simulink model "kinematics"  (R2019a)
settings: Solver=ode45  StartTime=0.0  StopTime=60  RelTol=2.8421709430404007E-14
undefined symbols (not defined in the file or in its folder): A0_BI, q0_BI, theta0_BI, wbi0_B, X, Y, Z, zyx0
libraries: sm_lib x3, nesl_utility x1
settings Model: Creator=bbingham  LastModifiedBy=tjones
settings DataIOCC: ReturnWorkspaceOutputs=off
settings DebuggingCC: ArithmeticOperatorsInVariantConditions=warning
settings SFSimCC: SimUseLocalCustomCode=off
settings RTWCC: SystemTargetFile=sldrt.tlc  TemplateMakefile=sldrt.tmf  Description=Simulink Desktop Real-Time  RTWUseLocalCustomCode=off  RTWCompilerOptimization=on
settings CodeAppCC: MaxIdLength=95  StateflowObjectComments=on
settings TargetCC: TargetPreCompLibLocation=C:\Program Files\MATLAB\R2019a\toolbox\sldrt\lib\win64  TargetLangStandard=C99 (ISO)  GeneratePreprocessorConditionals=Use local settings  SupportVariableSizeSignals=on  PreserveStateflowLocalDataDimensions=off

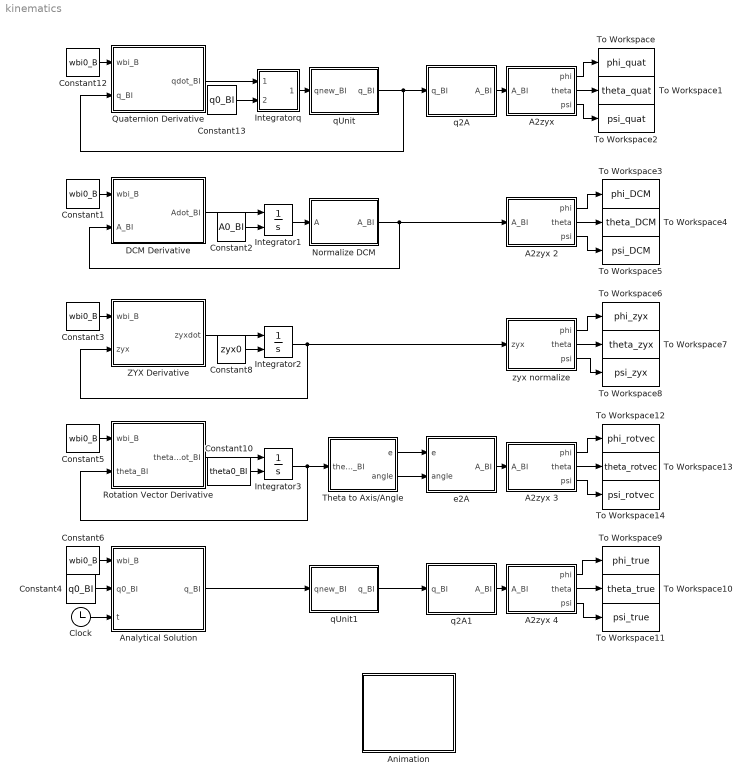
== system kinematics ==
  A2zyx : MATLAB Function  TreatAsAtomicUnit=on
  A2zyx 2 : MATLAB Function  TreatAsAtomicUnit=on
  A2zyx 3 : MATLAB Function  TreatAsAtomicUnit=on
  A2zyx 4 : MATLAB Function  TreatAsAtomicUnit=on
  Analytical Solution : MATLAB Function  TreatAsAtomicUnit=on
  Animation : Subsystem
  Clock : Clock
  Constant{1,3,5..6,12} (5 alike) : Constant  Value=wbi0_B
  Constant10 : Constant  Value=theta0_BI  VectorParams1D=off  SampleTime=0
  Constant13 : Constant  Value=q0_BI  OutDataTypeStr=Bus: qBus
  Constant2 : Constant  Value=A0_BI  VectorParams1D=off  SampleTime=0
  Constant4 : Constant  Value=q0_BI  VectorParams1D=off  OutDataTypeStr=Bus: qBus  SampleTime=0
  Constant8 : Constant  Value=zyx0  VectorParams1D=off  SampleTime=0
  DCM Derivative : MATLAB Function  TreatAsAtomicUnit=on
  Integrator1 : Integrator  InitialConditionSource=external
  Integrator2 : Integrator  InitialConditionSource=external
  Integrator3 : Integrator  InitialConditionSource=external
  Integratorq : Subsystem
  Normalize DCM : MATLAB Function  TreatAsAtomicUnit=on
  Quaternion Derivative : MATLAB Function  TreatAsAtomicUnit=on
  Rotation Vector Derivative : MATLAB Function  TreatAsAtomicUnit=on
  Theta to Axis/Angle : MATLAB Function  TreatAsAtomicUnit=on
  To Workspace : ToWorkspace  VariableName=phi_quat  SampleTime=-1
  To Workspace1 : ToWorkspace  VariableName=theta_quat  SampleTime=-1
  To Workspace10 : ToWorkspace  VariableName=theta_true  SampleTime=-1
  To Workspace11 : ToWorkspace  VariableName=psi_true  SampleTime=-1
  To Workspace12 : ToWorkspace  VariableName=phi_rotvec  SampleTime=-1
  To Workspace13 : ToWorkspace  VariableName=theta_rotvec  SampleTime=-1
  To Workspace14 : ToWorkspace  VariableName=psi_rotvec  SampleTime=-1
  To Workspace2 : ToWorkspace  VariableName=psi_quat  SampleTime=-1
  To Workspace3 : ToWorkspace  VariableName=phi_DCM  SampleTime=-1
  To Workspace4 : ToWorkspace  VariableName=theta_DCM  SampleTime=-1
  To Workspace5 : ToWorkspace  VariableName=psi_DCM  SampleTime=-1
  To Workspace6 : ToWorkspace  VariableName=phi_zyx  SampleTime=-1
  To Workspace7 : ToWorkspace  VariableName=theta_zyx  SampleTime=-1
  To Workspace8 : ToWorkspace  VariableName=psi_zyx  SampleTime=-1
  To Workspace9 : ToWorkspace  VariableName=phi_true  SampleTime=-1
  ZYX Derivative : MATLAB Function  TreatAsAtomicUnit=on
  e2A : MATLAB Function  TreatAsAtomicUnit=on
  q2A : MATLAB Function  TreatAsAtomicUnit=on
  q2A1 : MATLAB Function  TreatAsAtomicUnit=on
  qUnit : MATLAB Function  TreatAsAtomicUnit=on
  qUnit1 : MATLAB Function  TreatAsAtomicUnit=on
  zyx normalize : MATLAB Function  TreatAsAtomicUnit=on
  wires:
  Constant2/1 -> Integrator1/2
  DCM Derivative/1(Adot_BI) -> Integrator1/1
  Clock/1 -> Analytical Solution/3(t)
  Constant6/1 -> Analytical Solution/1(wbi_B)
  Constant1/1 -> DCM Derivative/1(wbi_B)
  Integrator1/1 -> Normalize DCM/1(A)
  q2A/1(A_BI) -> A2zyx/1(A_BI)
  A2zyx/2(theta) -> To Workspace1/1
  A2zyx/1(phi) -> To Workspace/1
  A2zyx/3(psi) -> To Workspace2/1
  q2A1/1(A_BI) -> A2zyx 4/1(A_BI)
  Analytical Solution/1(q_BI) -> qUnit1/1(qnew_BI)
  Constant3/1 -> ZYX Derivative/1(wbi_B)
  Constant8/1 -> Integrator2/2
  ZYX Derivative/1(zyxdot) -> Integrator2/1
  Integrator2/1 -> zyx normalize/1(zyx), ZYX Derivative/2(zyx)
  A2zyx 2/3(psi) -> To Workspace5/1
  A2zyx 2/1(phi) -> To Workspace3/1
  A2zyx 2/2(theta) -> To Workspace4/1
  zyx normalize/2(theta) -> To Workspace7/1
  zyx normalize/1(phi) -> To Workspace6/1
  zyx normalize/3(psi) -> To Workspace8/1
  A2zyx 4/3(psi) -> To Workspace11/1
  A2zyx 4/1(phi) -> To Workspace9/1
  A2zyx 4/2(theta) -> To Workspace10/1
  Normalize DCM/1(A_BI) -> A2zyx 2/1(A_BI), DCM Derivative/2(A_BI)
  A2zyx 3/3(psi) -> To Workspace14/1
  Rotation Vector Derivative/1(thetadot_BI) -> Integrator3/1
  A2zyx 3/1(phi) -> To Workspace12/1
  Constant10/1 -> Integrator3/2
  Integrator3/1 -> Rotation Vector Derivative/2(theta_BI), Theta to Axis/Angle/1(theta_BI)
  A2zyx 3/2(theta) -> To Workspace13/1
  Constant5/1 -> Rotation Vector Derivative/1(wbi_B)
  Theta to Axis/Angle/1(e) -> e2A/1(e)
  Theta to Axis/Angle/2(angle) -> e2A/2(angle)
  e2A/1(A_BI) -> A2zyx 3/1(A_BI)
  Constant4/1 -> Analytical Solution/2(q0_BI)
  Integratorq/1(qnew_BI) -> qUnit/1(qnew_BI)
  Constant12/1 -> Quaternion Derivative/1(wbi_B)
  Constant13/1 -> Integratorq/2(q0_BI)
  Quaternion Derivative/1(qdot_BI) -> Integratorq/1(qdot_BI)
  qUnit/1(q_BI) -> Quaternion Derivative/2(q_BI), q2A/1(q_BI)
  qUnit1/1(q_BI) -> q2A1/1(q_BI)

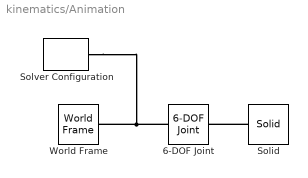
== system kinematics/Animation ==
  6-DOF Joint : sm_lib/Joints/6-DOF Joint  SenseConstraintForce=off  SenseConstraintForceX=off  SenseConstraintForceY=off  SenseConstraintForceZ=off  SenseConstraintTorque=off  SenseConstraintTorqueX=off  SenseConstraintTorqueY=off  SenseConstraintTorqueZ=off  SenseTotalForce=off  SenseTotalForceX=off  SenseTotalForceY=off  SenseTotalForceZ=off  SenseTotalTorque=off  SenseTotalTorqueX=off  SenseTotalTorqueY=off  SenseTotalTorqueZ=off  CompositeWrenchDir=FollowerOnBase  CompositeWrenchFrame=BaseFrame  PxEquilibriumPosition=0  PxEquilibriumPositionUnits=m  PxSpringStiffness=0  PxSpringStiffnessUnits=N/m  PxDampingCoefficient=0  PxDampingCoefficientUnits=N/(m/s)  PxTorqueActuationMode=NoTorque  PxMotionActuationMode=ComputedMotion  PxSensePosition=off  PxSenseVelocity=off  PxSenseAcceleration=off  PxSenseTorqueForce=off  PxSenseLowerLimitTorqueForce=off  PxSenseUpperLimitTorqueForce=off  PxLowerLimitSpecify=off  PxLowerLimitBound=-1  PxLowerLimitBoundUnits=m  PxLowerLimitStiffness=1e6  PxLowerLimitStiffnessUnits=N/m  PxLowerLimitDamping=1e3  PxLowerLimitDampingUnits=N/(m/s)  PxLowerLimitTransitionRegionWidth=1e-4  PxLowerLimitTransitionRegionWidthUnits=m  PxUpperLimitSpecify=off  PxUpperLimitBound=1  PxUpperLimitBoundUnits=m  PxUpperLimitStiffness=1e6  PxUpperLimitStiffnessUnits=N/m  PxUpperLimitDamping=1e3  PxUpperLimitDampingUnits=N/(m/s)  PxUpperLimitTransitionRegionWidth=1e-4  PxUpperLimitTransitionRegionWidthUnits=m  PxPositionTargetSpecify=off  PxPositionTargetPriority=High  PxPositionTargetValue=0  PxPositionTargetValueUnits=m  PxVelocityTargetSpecify=off  PxVelocityTargetPriority=High  PxVelocityTargetValue=0  PxVelocityTargetValueUnits=m/s  PyEquilibriumPosition=0  PyEquilibriumPositionUnits=m  PySpringStiffness=0  PySpringStiffnessUnits=N/m  PyDampingCoefficient=0  PyDampingCoefficientUnits=N/(m/s)  PyTorqueActuationMode=NoTorque  PyMotionActuationMode=ComputedMotion  PySensePosition=off  PySenseVelocity=off  PySenseAcceleration=off  PySenseTorqueForce=off  PySenseLowerLimitTorqueForce=off  PySenseUpperLimitTorqueForce=off  PyLowerLimitSpecify=off  PyLowerLimitBound=-1  PyLowerLimitBoundUnits=m  PyLowerLimitStiffness=1e6  PyLowerLimitStiffnessUnits=N/m  PyLowerLimitDamping=1e3  PyLowerLimitDampingUnits=N/(m/s)  PyLowerLimitTransitionRegionWidth=1e-4  PyLowerLimitTransitionRegionWidthUnits=m  PyUpperLimitSpecify=off  PyUpperLimitBound=1  PyUpperLimitBoundUnits=m  PyUpperLimitStiffness=1e6  PyUpperLimitStiffnessUnits=N/m  PyUpperLimitDamping=1e3  PyUpperLimitDampingUnits=N/(m/s)  PyUpperLimitTransitionRegionWidth=1e-4  PyUpperLimitTransitionRegionWidthUnits=m  PyPositionTargetSpecify=off  PyPositionTargetPriority=High  PyPositionTargetValue=0  PyPositionTargetValueUnits=m  PyVelocityTargetSpecify=off  PyVelocityTargetPriority=High  PyVelocityTargetValue=0  PyVelocityTargetValueUnits=m/s  PzEquilibriumPosition=0  PzEquilibriumPositionUnits=m  PzSpringStiffness=0  PzSpringStiffnessUnits=N/m  PzDampingCoefficient=0  PzDampingCoefficientUnits=N/(m/s)  PzTorqueActuationMode=NoTorque  PzMotionActuationMode=ComputedMotion  PzSensePosition=off  PzSenseVelocity=off  PzSenseAcceleration=off  PzSenseTorqueForce=off  PzSenseLowerLimitTorqueForce=off  PzSenseUpperLimitTorqueForce=off  PzLowerLimitSpecify=off  PzLowerLimitBound=-1  PzLowerLimitBoundUnits=m  PzLowerLimitStiffness=1e6  PzLowerLimitStiffnessUnits=N/m  PzLowerLimitDamping=1e3  PzLowerLimitDampingUnits=N/(m/s)  PzLowerLimitTransitionRegionWidth=1e-4  PzLowerLimitTransitionRegionWidthUnits=m  PzUpperLimitSpecify=off  PzUpperLimitBound=1  PzUpperLimitBoundUnits=m  PzUpperLimitStiffness=1e6  PzUpperLimitStiffnessUnits=N/m  PzUpperLimitDamping=1e3  PzUpperLimitDampingUnits=N/(m/s)  PzUpperLimitTransitionRegionWidth=1e-4  PzUpperLimitTransitionRegionWidthUnits=m  PzPositionTargetSpecify=off  PzPositionTargetPriority=High  PzPositionTargetValue=0  PzPositionTargetValueUnits=m  PzVelocityTargetSpecify=off  PzVelocityTargetPriority=High  PzVelocityTargetValue=0  PzVelocityTargetValueUnits=m/s  SphDefPosRotationMethod=None  SphDefPosRotationAngleUnits=deg  SphDefPosRotationStandardAxis=+Z  SphDefPosRotationAngle=0.0  SphDefPosRotationArbitraryAxis=[0 0 1]  SphDefPosFollAlignAxisA=+X  SphDefPosBaseAlignAxisA=+Y  SphDefPosFollAlignAxisB=+Y  SphDefPosBaseAlignAxisB=+Z  SphDefPosRotationSequenceAxes=FollowerAxes  SphDefPosRotationSequence=XYX  SphDefPosRotationSequenceAngles=[0 0 0]  SphDefPosRotationSequenceAnglesUnits=deg  SphDefPosRotationMatrix=[1 0 0; 0 1 0; 0 0 1]  SphEqPosRotationMethod=None  SphEqPosRotationAngleUnits=deg  SphEqPosRotationStandardAxis=+Z  SphEqPosRotationAngle=0.0  SphEqPosRotationArbitraryAxis=[0 0 1]  SphEqPosFollAlignAxisA=+X  SphEqPosBaseAlignAxisA=+Y  SphEqPosFollAlignAxisB=+Y  SphEqPosBaseAlignAxisB=+Z  SphEqPosRotationSequenceAxes=FollowerAxes  SphEqPosRotationSequence=XYX  SphEqPosRotationSequenceAngles=[0 0 0]  SphEqPosRotationSequenceAnglesUnits=deg  SphEqPosRotationMatrix=[1 0 0; 0 1 0; 0 0 1]  SphSpringStiffness=0  SphSpringStiffnessUnits=N*m/deg  SphDampingCoefficient=0  SphDampingCoefficientUnits=N*m/(deg/s)  SphActuateTorqueX=off  SphActuateTorqueY=off  SphActuateTorqueZ=off  SphActuateTorque=off  SphTorqueActuationMode=NoTorque  SphMotionActuationMode=ComputedMotion  SphActuationFrame=BaseFrame  SphSensePosition=off  SphSenseVelocityX=off  SphSenseVelocityY=off  SphSenseVelocityZ=off  SphSenseVelocity=off  SphSenseAccelerationX=off  SphSenseAccelerationY=off  SphSenseAccelerationZ=off  SphSenseAcceleration=off  SphSenseTorqueX=off  SphSenseTorqueY=off  SphSenseTorqueZ=off  SphSenseTorqueForce=off  SphSenseLowerLimitTorqueMag=off  SphSenseUpperLimitTorqueMag=off  SphSensingFrame=BaseFrame  SphLowerLimitSpecify=off  SphLowerLimitBound=15  SphLowerLimitBoundUnits=deg  SphLowerLimitStiffness=1e4  SphLowerLimitStiffnessUnits=N*m/deg  SphLowerLimitDamping=10  SphLowerLimitDampingUnits=N*m/(deg/s)  SphLowerLimitTransitionRegionWidth=0.1  SphLowerLimitTransitionRegionWidthUnits=deg  SphUpperLimitSpecify=off  SphUpperLimitBound=45  SphUpperLimitBoundUnits=deg  SphUpperLimitStiffness=1e4  SphUpperLimitStiffnessUnits=N*m/deg  SphUpperLimitDamping=10  SphUpperLimitDampingUnits=N*m/(deg/s)  SphUpperLimitTransitionRegionWidth=0.1  SphUpperLimitTransitionRegionWidthUnits=deg  SphPositionTargetRotationMethod=None  SphPositionTargetRotationAngleUnits=deg  SphPositionTargetRotationStandardAxis=+Z  SphPositionTargetRotationAngle=0.0  SphPositionTargetRotationArbitraryAxis=[0 0 1]  SphPositionTargetFollAlignAxisA=+X  SphPositionTargetBaseAlignAxisA=+Y  SphPositionTargetFollAlignAxisB=+Y  SphPositionTargetBaseAlignAxisB=+Z  SphPositionTargetRotationSequenceAxes=FollowerAxes  SphPositionTargetRotationSequence=XYX  SphPositionTargetRotationSequenceAngles=[0 0 0]  SphPositionTargetRotationSequenceAnglesUnits=deg  SphPositionTargetRotationMatrix=[1 0 0; 0 1 0; 0 0 1]  SphPositionTargetSpecify=off  SphPositionTargetPriority=High  SphVelocityTargetValue=wbi0_B  SphVelocityTargetValueUnits=rad/s  SphVelocityTargetSpecify=on  SphVelocityTargetPriority=High  SphVelocityTargetInFollowerFrame=on
  Solid : sm_lib/Body Elements/Solid  InertiaType=CalculateFromGeometry  Mass=1  MassUnits=kg  CenterOfMass=[0 0 0]  CenterOfMassUnits=m  MomentsOfInertia=[1 1 1]  MomentsOfInertiaUnits=kg*m^2  ProductsOfInertia=[0 0 0]  ProductsOfInertiaUnits=kg*m^2  BasedOnType=Density  Density=1000  DensityUnits=kg/m^3  DoExposeReferenceFrame=on  SerializedFrames=<Frames/>  GraphicType=FromGeometry  MarkerShape=Sphere  MarkerSize=10  GraphicVisPropType=SimpleVisualProperties  GraphicDiffuseColor=[0.8 1.0 1.0]  GraphicSpecularColor=[0.5 0.5 0.5 1.0]  GraphicAmbientColor=[0.15 0.15 0.15 1.0]  GraphicEmissiveColor=[0.0 0.0 0.0 1.0]  GraphicShininess=75  GraphicOpacity=1.0  GeometryShape=Brick  RectangleSize=[1 1]  RectangleSizeUnits=m  BrickDimensions=[1 2 3]  BrickDimensionUnits=m  CylinderRadius=1  CylinderRadiusUnits=m  CylinderLength=1  CylinderLengthUnits=m  SphereRadius=1  SphereRadiusUnits=m  EllipsoidRadii=[1 1 1]  EllipsoidRadiiUnits=m  ExtrusionCrossSection=[1 1; -1 1; -1 -1; 1 -1]  ExtrusionCrossSectionUnits=m  ExtrusionLength=1  ExtrusionLengthUnits=m  PolygonNumSides=3  PolygonOuterRadius=1  PolygonOuterRadiusUnits=m  ExtGeomFileType=STEP  ExtGeomFileUnits=m  RevolutionCrossSection=[1 1; 1 -1; 2 -1; 2 1]  RevolutionCrossSectionUnits=m  RevolutionExtent=Full  RevolutionAngle=180  RevolutionAngleUnits=deg
  Solver Configuration : nesl_utility/Solver Configuration  PhysicalDomain=network_engine_domain  SubClassName=solver  LeftPortType=input  RightPortType=generic  Tones=[]  Harmonics=[]  SimulateNoise=off  Profile=off  UseLocalSampling=off  EnableSwitchedLinearOptims=on  FrequencyDomain=off  UseCCode=off  RelTol=0.001  AbsTol=1e-06  MinStep=1e-09  ToWorkspace=off  RevertToSquareIcSolve=off  NumHomotopyIterations=100  PhasorMode=off  PhasorModeNumHarmonics=1  DoDC=off  ResidualTolerance=1e-09  UseLocalSolver=off  LocalSolverChoice=NE_BACKWARD_EULER_ADVANCER  LocalSolverSampleTime=0.001  DoFixedCost=off  MaxNonlinIter=3  MaxModeIter=2  LinearAlgebra=auto  EquationFormulation=NE_TIME_EF  DelaysMemoryBudget=1024  AutomaticFiltering=on  FilteringTimeConstant=0.001  PartitionStorageMethod=AS_NEEDED  PartitionMemoryBudget=1024  PartitionMethod=ROBUST
  World Frame : sm_lib/Frames and Transforms/World Frame
  connections:
  6-DOF Joint/LConn1 -- Solver Configuration/RConn1 -- World Frame/RConn1
  Solid/RConn1 -- 6-DOF Joint/RConn1

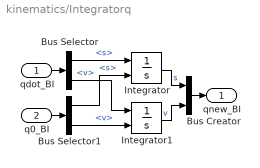
== system kinematics/Integratorq ==
  qdot_BI : Inport  OutDataTypeStr=Bus: qBus
  q0_BI : Inport  Port=2  OutDataTypeStr=Bus: qBus
  Bus Creator : BusCreator  Inputs=2  OutDataTypeStr=Bus: qBus
      settings: InheritFromInputs=off
  Bus Selector : BusSelector  OutputSignals=s,v
  Bus Selector1 : BusSelector  OutputSignals=s,v
  Integrator : Integrator  InitialConditionSource=external
  Integrator1 : Integrator  InitialConditionSource=external
  qnew_BI : Outport  OutDataTypeStr=Bus: qBus
  wires:
  qdot_BI/1 -> Bus Selector/1
  q0_BI/1 -> Bus Selector1/1
  Bus Selector/1 -> Integrator/1  "<s>"
  Bus Selector1/1 -> Integrator/2  "<s>"
  Bus Selector/2 -> Integrator1/1  "<v>"
  Bus Selector1/2 -> Integrator1/2  "<v>"
  Integrator/1 -> Bus Creator/1  "s"
  Integrator1/1 -> Bus Creator/2  "v"
  Bus Creator/1 -> qnew_BI/1

== matlab function kinematics/Analytical Solution ==
  data: wbi_B input; q0_BI input Bus: qBus; q_BI output Bus: qBus; t input
function q_BI = fcn(wbi_B, q0_BI, t)

norm_w = norm(wbi_B);
if (norm_w == 0)
    q_BI.s = q0_BI.s;
    q_BI.v = q0_BI.v;
else
    c = cos(1/2*norm_w*t);
    psi = sin(1/2*norm_w*t)*wbi_B/norm_w;

    q_BI.s = c*q0_BI.s - psi'*q0_BI.v;
    q_BI.v = q0_BI.s*psi + c*q0_BI.v - X(psi)*q0_BI.v;
end

== matlab function kinematics/DCM Derivative ==
  data: wbi_B input; A_BI input; Adot_BI output
function Adot_BI = fcn(wbi_B, A_BI)

Adot_BI = -1 * X(wbi_B) * A_BI;

== matlab function kinematics/Quaternion Derivative ==
  data: wbi_B input; q_BI input Bus: qBus; qdot_BI output Bus: qBus
function qdot_BI = fcn(wbi_B, q_BI)

w.s = 0;
w.v = wbi_B;

qdot = qX(w, q_BI);

qdot_BI.s = 1/2*qdot.s;
qdot_BI.v = 1/2*qdot.v;

== matlab function kinematics/A2zyx 2 ==
  data: A_BI input; phi output; theta output; psi output
function [phi,theta,psi] = fcn(A_BI)

[phi, theta, psi] = A2zyx(A_BI);

== matlab function kinematics/qUnit1 ==
  data: qnew_BI input Bus: qBus; q_BI output Bus: qBus
function q_BI = fcn(qnew_BI)

q_BI = qUnit(qnew_BI);

== matlab function kinematics/q2A ==
  data: q_BI input Bus: qBus; A_BI output
function A_BI = fcn(q_BI)

A_BI = q2A(q_BI);

== matlab function kinematics/A2zyx ==
  data: A_BI input; phi output; theta output; psi output
function [phi,theta,psi] = fcn(A_BI)

[phi, theta, psi] = A2zyx(A_BI);

== matlab function kinematics/q2A1 ==
  data: q_BI input Bus: qBus; A_BI output
function A_BI = fcn(q_BI)

A_BI = q2A(q_BI);

== matlab function kinematics/A2zyx 3 ==
  data: A_BI input; phi output; theta output; psi output
function [phi,theta,psi] = fcn(A_BI)

[phi, theta, psi] = A2zyx(A_BI);

== matlab function kinematics/ZYX Derivative ==
  data: wbi_B input; zyx input; zyxdot output
function zyxdot = fcn(wbi_B, zyx)

cth = cos(zyx(2));
sth = sin(zyx(2));
sps = sin(zyx(3));
cps = cos(zyx(3));
B = 1/cth * [0, sps, cps; 0, cth*cps, -1*cth*sps; cth, sth*sps, sth*cps];
zyxdot = B * wbi_B;

== matlab function kinematics/zyx normalize ==
  data: zyx input; phi output; theta output; psi output
function [phi,theta,psi] = fcn(zyx)

A_BI = euler2A(3,2,1,zyx(1),zyx(2),zyx(3));

[phi,theta,psi] = A2zyx(A_BI);

== matlab function kinematics/Normalize DCM ==
  data: A input; A_BI output
function A_BI = fcn(A)

E = 1/2*(A*A'-eye(3));
A_BI = (eye(3)-E)*A;

== matlab function kinematics/Rotation Vector Derivative ==
  data: wbi_B input; theta_BI input; thetadot_BI output
function thetadot_BI = fcn(wbi_B, theta_BI)

th_X = X(theta_BI);
th_M = norm(theta_BI);
term3 = 1/(th_M^2) * (1 - th_M/2 * cot(th_M/2)) * th_X * (th_X * wbi_B);
thetadot_BI = wbi_B + 1/2*th_X*wbi_B + term3;

== matlab function kinematics/Theta to Axis//Angle ==
  data: theta_BI input; e output; angle output
function [e, angle] = fcn(theta_BI)

angle = norm(theta_BI);

if(angle == 0)
    e = [1; 0; 0];
else
    e = theta_BI/angle;
end

== matlab function kinematics/e2A ==
  data: e input; A_BI output; angle input
function A_BI = fcn(e, angle)

A_BI = e2A(e,angle);

== matlab function kinematics/A2zyx 4 ==
  data: A_BI input; phi output; theta output; psi output
function [phi,theta,psi] = fcn(A_BI)

[phi, theta, psi] = A2zyx(A_BI);

== matlab function kinematics/qUnit ==
  data: qnew_BI input Bus: qBus; q_BI output Bus: qBus
function q_BI = fcn(qnew_BI)

q_BI = qUnit(qnew_BI);
